simulink model "lista2_item_e"  (R2014b)
settings: Solver=ode45  StartTime=0.0  StopTime=Tsim  RelTol=1e-3
values from neighbouring files (symbols this model uses):
  T = 1    [sistema_lista2.m]
settings Model: Creator=Danilo  LastModifiedBy=Danilo

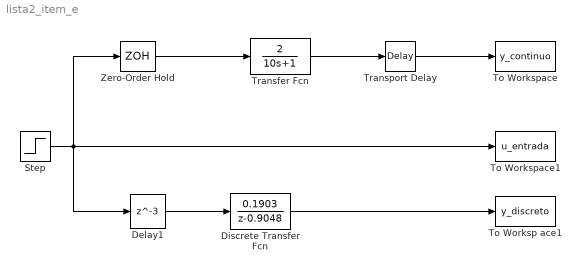
== system lista2_item_e ==
  Delay1 : Delay  DelayLength=3  SampleTime=T
  Discrete Transfer Fcn : DiscreteTransferFcn  Numerator=[0.1903]  Denominator=[1 -0.9048]  SampleTime=T
  Step : Step  Time=0  After=0.1  SampleTime=T
  To Worksp ace1 : ToWorkspace  VariableName=y_discreto  SampleTime=T
  To Workspace : ToWorkspace  VariableName=y_continuo  SampleTime=T
  To Workspace1 : ToWorkspace  VariableName=u_entrada  SampleTime=T
  Transfer Fcn : TransferFcn  Numerator=2  Denominator=[10 1]
  Transport Delay : TransportDelay  DelayTime=3
  Zero-Order Hold : ZeroOrderHold  SampleTime=T
  wires:
  Step/1 -> Delay1/1, Zero-Order Hold/1, To Workspace1/1
  Discrete Transfer Fcn/1 -> To Worksp ace1/1
  Transfer Fcn/1 -> Transport Delay/1
  Zero-Order Hold/1 -> Transfer Fcn/1
  Transport Delay/1 -> To Workspace/1
  Delay1/1 -> Discrete Transfer Fcn/1
